simulink model "UAV_MPC_Tracking3D"  (R2025b)
settings: Solver=FixedStepDiscrete  StartTime=0.0  StopTime=29.9  FixedStep=Ts  RelTol=1e-3
InitFcn:
  | % Load controller matrices
  | load('data/mpcController3D.mat');   % loads Ad, Bd, mpcObj3D
  | 
  | % Load multi-UAV missions
  | load('data/MultiUAV_References.mat');  % loads missions, Ts
  | 
  | % Create reference timeseries for each UAV
  | refTS1 = missions(1).refTS;
  | refTS2 = missions(2).refTS;
  | refTS3 = missions(3).refTS;
  | refTS4 = missions(4).refTS;
undefined symbols (not defined in the file): Ad, Bd, Ts
libraries: mpclib x4, simulink x1
settings Model: Creator=EBIRON  LastModifiedBy=Lenovo

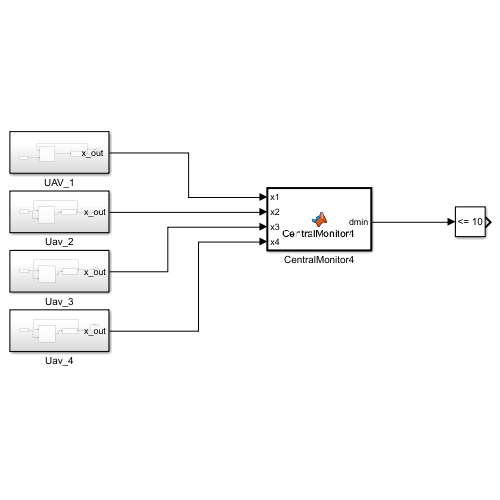
[thumbnail: Simulink's stored preview of the top-level diagram]
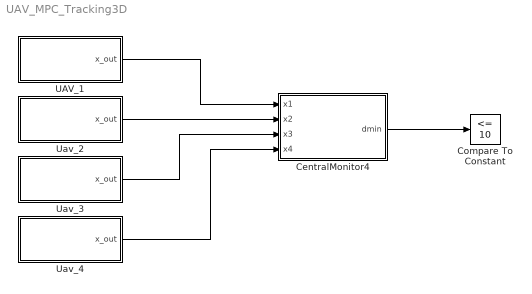
== system UAV_MPC_Tracking3D ==
  "CentralMonitor4 " : MATLAB Function  TreatAsAtomicUnit=on
  Compare To Constant : simulink/Logic and Bit Operations/Compare To Constant  relop=<=  const=10  OutDataTypeStr=boolean
  UAV_1 : Subsystem
  Uav_2 : Subsystem
  Uav_3 : Subsystem
  Uav_4 : Subsystem
  wires:
  "CentralMonitor4 "/1(dmin) -> Compare To Constant/1
  UAV_1/1("x_out ") -> "CentralMonitor4 "/1(x1)
  Uav_2/1(x_out) -> "CentralMonitor4 "/2(x2)
  Uav_3/1(x_out) -> "CentralMonitor4 "/3(x3)
  Uav_4/1(x_out) -> "CentralMonitor4 "/4(x4)

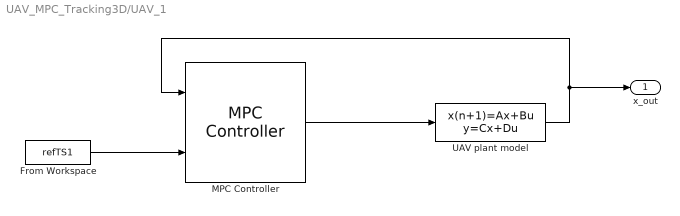
== system UAV_MPC_Tracking3D/UAV_1 ==
  From Workspace : FromWorkspace  VariableName=refTS1  SampleTime=Ts  OutputAfterFinalValue=Holding final value
  MPC Controller : mpclib/MPC Controller  SCDEnableBlockLinearizationSpecification=on  mpcobj=mpcObj3D  is_multiple=0  enable_value=0  return_u0=off  updateMPCinCallerWorkspace=on  md_inport=off  mv_inport=off  uref_inport=off  return_cost=off  return_mvseq=off  return_qpstatus=off  return_xseq=off  return_state=off  return_ovseq=off  state_inport=off  umin_inport=off  umax_inport=off  ymin_inport=off  ymax_inport=off  cc_inport=off  ywt_inport=off  uwt_inport=off  duwt_inport=off  rhoeps_inport=off  pm_inport=off  MaximumP=10  HorizonChoice=FixedHorizon  n_ts=0.1  n_p=40  n_mv=3  n_md=0  n_ud=0  n_mo=6  n_uo=0  BlockDataType=double  SampleTimeInherited=off  switch_inport=off
  UAV plant model : DiscreteStateSpace  A=Ad  B=Bd  C=eye(6)  D=zeros(6,3)  InitialCondition=refTS1.Data(1,:)'  SampleTime=Ts
  "x_out " : Outport
  wires:
  MPC Controller/1 -> UAV plant model/1
  UAV plant model/1 -> MPC Controller/1, "x_out "/1
  From Workspace/1 -> MPC Controller/2

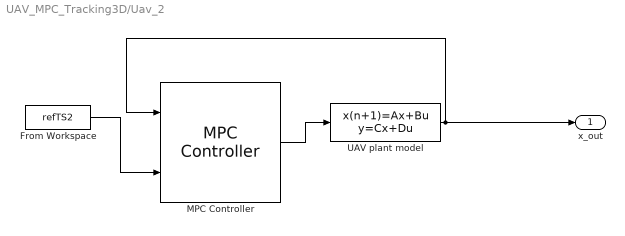
== system UAV_MPC_Tracking3D/Uav_2 ==
  From Workspace : FromWorkspace  VariableName=refTS2  SampleTime=Ts  OutputAfterFinalValue=Holding final value
  MPC Controller : mpclib/MPC Controller  SCDEnableBlockLinearizationSpecification=on  mpcobj=mpcObj3D  is_multiple=0  enable_value=0  return_u0=off  updateMPCinCallerWorkspace=on  md_inport=off  mv_inport=off  uref_inport=off  return_cost=off  return_mvseq=off  return_qpstatus=off  return_xseq=off  return_state=off  return_ovseq=off  state_inport=off  umin_inport=off  umax_inport=off  ymin_inport=off  ymax_inport=off  cc_inport=off  ywt_inport=off  uwt_inport=off  duwt_inport=off  rhoeps_inport=off  pm_inport=off  MaximumP=10  HorizonChoice=FixedHorizon  n_ts=0.1  n_p=40  n_mv=3  n_md=0  n_ud=0  n_mo=6  n_uo=0  BlockDataType=double  SampleTimeInherited=off  switch_inport=off
  UAV plant model : DiscreteStateSpace  A=Ad  B=Bd  C=eye(6)  D=zeros(6,3)  InitialCondition=refTS2.Data(1,:)'  SampleTime=Ts
  x_out : Outport
  wires:
  UAV plant model/1 -> MPC Controller/1, x_out/1
  From Workspace/1 -> MPC Controller/2
  MPC Controller/1 -> UAV plant model/1

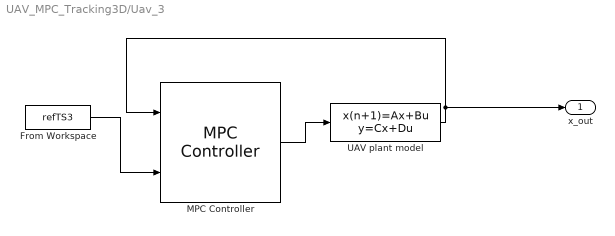
== system UAV_MPC_Tracking3D/Uav_3 ==
  From Workspace : FromWorkspace  VariableName=refTS3  SampleTime=Ts  OutputAfterFinalValue=Holding final value
  MPC Controller : mpclib/MPC Controller  SCDEnableBlockLinearizationSpecification=on  mpcobj=mpcObj3D  is_multiple=0  enable_value=0  return_u0=off  updateMPCinCallerWorkspace=on  md_inport=off  mv_inport=off  uref_inport=off  return_cost=off  return_mvseq=off  return_qpstatus=off  return_xseq=off  return_state=off  return_ovseq=off  state_inport=off  umin_inport=off  umax_inport=off  ymin_inport=off  ymax_inport=off  cc_inport=off  ywt_inport=off  uwt_inport=off  duwt_inport=off  rhoeps_inport=off  pm_inport=off  MaximumP=10  HorizonChoice=FixedHorizon  n_ts=0.1  n_p=40  n_mv=3  n_md=0  n_ud=0  n_mo=6  n_uo=0  BlockDataType=double  SampleTimeInherited=off  switch_inport=off
  UAV plant model : DiscreteStateSpace  A=Ad  B=Bd  C=eye(6)  D=zeros(6,3)  InitialCondition=refTS3.Data(1,:)'  SampleTime=Ts
  x_out : Outport
  wires:
  UAV plant model/1 -> MPC Controller/1, x_out/1
  From Workspace/1 -> MPC Controller/2
  MPC Controller/1 -> UAV plant model/1

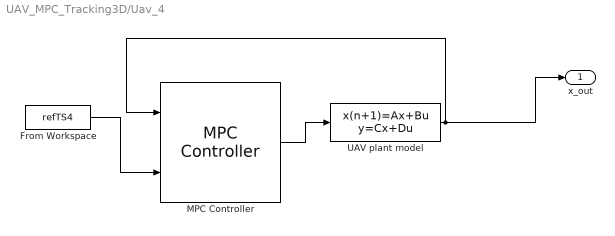
== system UAV_MPC_Tracking3D/Uav_4 ==
  From Workspace : FromWorkspace  VariableName=refTS4  SampleTime=Ts  OutputAfterFinalValue=Holding final value
  MPC Controller : mpclib/MPC Controller  SCDEnableBlockLinearizationSpecification=on  mpcobj=mpcObj3D  is_multiple=0  enable_value=0  return_u0=off  updateMPCinCallerWorkspace=on  md_inport=off  mv_inport=off  uref_inport=off  return_cost=off  return_mvseq=off  return_qpstatus=off  return_xseq=off  return_state=off  return_ovseq=off  state_inport=off  umin_inport=off  umax_inport=off  ymin_inport=off  ymax_inport=off  cc_inport=off  ywt_inport=off  uwt_inport=off  duwt_inport=off  rhoeps_inport=off  pm_inport=off  MaximumP=10  HorizonChoice=FixedHorizon  n_ts=0.1  n_p=40  n_mv=3  n_md=0  n_ud=0  n_mo=6  n_uo=0  BlockDataType=double  SampleTimeInherited=off  switch_inport=off
  UAV plant model : DiscreteStateSpace  A=Ad  B=Bd  C=eye(6)  D=zeros(6,3)  InitialCondition=refTS4.Data(1,:)'  SampleTime=Ts
  x_out : Outport
  wires:
  UAV plant model/1 -> MPC Controller/1, x_out/1
  From Workspace/1 -> MPC Controller/2
  MPC Controller/1 -> UAV plant model/1

== matlab function UAV_MPC_Tracking3D/CentralMonitor4  ==
  data: x1 input; dmin output; x2 input; x3 input; x4 input
function dmin = CentralMonitor4(x1,x2,x3,x4)

p1 = x1(1:3);
p2 = x2(1:3);
p3 = x3(1:3);
p4 = x4(1:3);

d12 = norm(p1-p2);
d13 = norm(p1-p3);
d14 = norm(p1-p4);
d23 = norm(p2-p3);
d24 = norm(p2-p4);
d34 = norm(p3-p4);

dmin = min([d12 d13 d14 d23 d24 d34]);

end
